simulink model "uuvSim_ampc"  (R2017b)
settings: Solver=ode4  StartTime=0.0  StopTime=10.0  FixedStep=mdl.tStep  RelTol=1e-3
values from neighbouring files (symbols this model uses):
  dt = block.DialogPrm(4).Data    [trj_gen.m]    (also in trj_gen_mpc.m; trj_mpc.m = block.DialogPrm(2).Data)
  p = block.DialogPrm(5).Data    [trj_gen_mpc.m]    (also in trj_mpc.m = block.DialogPrm(3).Data)
  trj = trj.trajectory_generation(block.CurrentTime)    [trj_gen.m]    (also in trj_gen_mpc.m = trj.trajectory_generation(block.CurrentTime+(i-1)*dt); trj_mpc.m = get_param(block.BlockHandle, 'UserData'))
undefined symbols (not defined in the file or in its folder): A, Ad, B, Bd, C, Cd, D, Dd, DX, ics, rov, Tinv, U, v_c, X, Y
libraries: mpclib x1
settings Model: Creator=e_anderlini  LastModifiedBy=e_anderlini
settings CodeAppCC: StateflowObjectComments=on

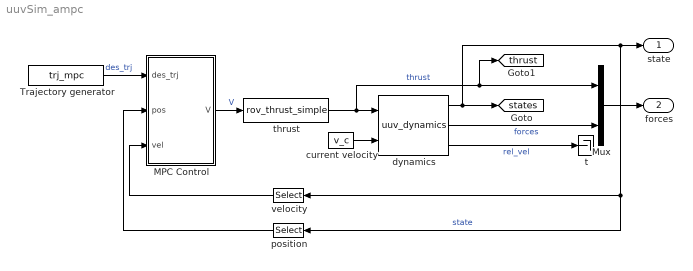
== system uuvSim_ampc ==
  MPC Control : Subsystem
  Mux : Mux  Inputs=[6,18]
  Trajectory generator : M-S-Function  FunctionName=trj_mpc  Parameters=trj,dt,p
  current velocity : Constant  Value=v_c
  dynamics : S-Function  FunctionName=uuv_dynamics  Parameters=rov.weight,rov.buoyancy,rov.CoG,rov.CoB,ics,rov.inv_mass',rov.M_A',rov.M_B',rov.D_l',rov.D_q'  SFunctionDeploymentMode=off  EnableBusSupport=off
  position : Selector  InputPortWidth=12  IndexOptions=Index vector (dialog)  Indices=[1 2 3 6]  OutputSizes=1
  t : Terminator
  thrust : S-Function  FunctionName=rov_thrust_simple  Parameters=rov.coeffs',rov.T'  SFunctionDeploymentMode=off  EnableBusSupport=off
  velocity : Selector  InputPortWidth=12  IndexOptions=Index vector (dialog)  Indices=[7 8 9 12]  OutputSizes=1
  state : Outport
  forces : Outport  Port=2
  tag scope: states=global, thrust=global
  wires:
  dynamics/1 -> [states], position/1, velocity/1, state/1  "state"
  thrust/1 -> [thrust], Mux/1, dynamics/1  "thrust"
  Mux/1 -> forces/1
  dynamics/2 -> Mux/2  "forces"
  MPC Control/1(V) -> thrust/1  "V"
  dynamics/3 -> t/1  "rel_vel"
  current velocity/1 -> dynamics/2
  position/1 -> MPC Control/2(pos)
  Trajectory generator/1 -> MPC Control/1(des_trj)  "des_trj"
  velocity/1 -> MPC Control/3(vel)

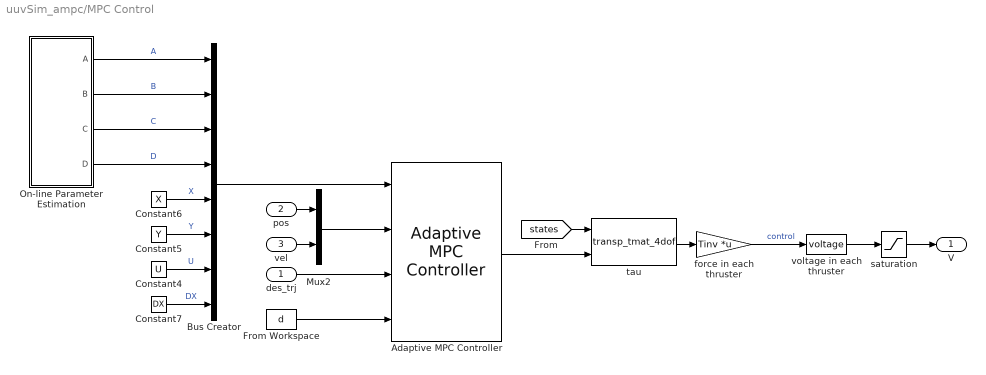
== system uuvSim_ampc/MPC Control ==
  des_trj : Inport
  pos : Inport  Port=2
  vel : Inport  Port=3
  Adaptive MPC Controller : mpclib/Adaptive MPC Controller  SCDEnableBlockLinearizationSpecification=on  mpcobj=mpc_kaxan  md_inport=on  mv_inport=off  cost_outport=off  return_sequence=off  return_qpstatus=off  return_state=off  state_inport=off  isltv_plant=off  lims_inport=off  cc_inport=off  ywt_inport=off  uwt_inport=off  duwt_inport=off  rhoeps_inport=off  uref_inport=off  BlockDataType=double  SampleTimeInherited=off  switch_inport=off
      settings: SourceProductName=Model Predictive Control Toolbox
  Bus Creator : BusCreator  Inputs=8
  Constant4 : Constant  Value=U  VectorParams1D=off
  Constant5 : Constant  Value=Y  VectorParams1D=off
  Constant6 : Constant  Value=X  VectorParams1D=off
  Constant7 : Constant  Value=DX  VectorParams1D=off
  From Workspace : FromWorkspace  VariableName=d  SampleTime=0
  Mux2 : Mux  Inputs=2
  On-line Parameter Estimation : Subsystem
  force in each thruster : Gain  Gain=Tinv  Multiplication=Matrix(K*u)
  saturation : Saturate  UpperLimit=5  LowerLimit=-5
  tau : S-Function  FunctionName=transp_tmat_4dof  SFunctionDeploymentMode=off  EnableBusSupport=off
  voltage in each thruster : S-Function  FunctionName=voltage  Parameters=rov.inv_coeffs'  SFunctionDeploymentMode=off  EnableBusSupport=off
  V : Outport
  wires:
  force in each thruster/1 -> voltage in each thruster/1  "control"
  saturation/1 -> V/1
  Adaptive MPC Controller/1 -> tau/2
  pos/1 -> Mux2/1
  [states] -> tau/1
  tau/1 -> force in each thruster/1
  voltage in each thruster/1 -> saturation/1
  vel/1 -> Mux2/2
  des_trj/1 -> Adaptive MPC Controller/3
  Mux2/1 -> Adaptive MPC Controller/2
  Bus Creator/1 -> Adaptive MPC Controller/1
  Constant7/1 -> Bus Creator/8  "DX"
  Constant4/1 -> Bus Creator/7  "U"
  Constant5/1 -> Bus Creator/6  "Y"
  Constant6/1 -> Bus Creator/5  "X"
  On-line Parameter Estimation/1(A) -> Bus Creator/1  "A"
  On-line Parameter Estimation/2(B) -> Bus Creator/2  "B"
  On-line Parameter Estimation/3(C) -> Bus Creator/3  "C"
  On-line Parameter Estimation/4(D) -> Bus Creator/4  "D"
  From Workspace/1 -> Adaptive MPC Controller/4

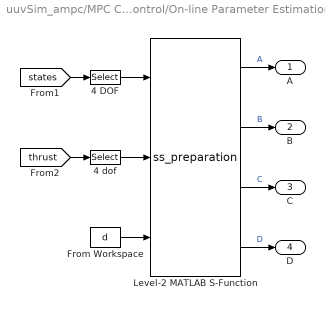
== system uuvSim_ampc/MPC Control/On-line Parameter Estimation ==
  4 DOF : Selector  InputPortWidth=12  IndexOptions=Index vector (dialog)  Indices=[1 2 3 6 7 8 9 12]  OutputSizes=1
  4 dof : Selector  InputPortWidth=6  IndexOptions=Index vector (dialog)  Indices=[1 2 3 6]  OutputSizes=1
  From Workspace : FromWorkspace  VariableName=d  SampleTime=0
  Level-2 MATLAB S-Function : M-S-Function  FunctionName=ss_preparation  Parameters=Ad,Bd,Cd,Dd,A,B,C,D
  A : Outport
  B : Outport  Port=2
  C : Outport  Port=3
  D : Outport  Port=4
  wires:
  4 DOF/1 -> Level-2 MATLAB S-Function/1
  [states] -> 4 DOF/1
  [thrust] -> 4 dof/1
  Level-2 MATLAB S-Function/1 -> A/1  "A"
  Level-2 MATLAB S-Function/3 -> C/1  "C"
  Level-2 MATLAB S-Function/2 -> B/1  "B"
  Level-2 MATLAB S-Function/4 -> D/1  "D"
  4 dof/1 -> Level-2 MATLAB S-Function/2
  From Workspace/1 -> Level-2 MATLAB S-Function/3
